simulink model "Q1b_Half_Controlled"  (R2018a)
settings: Solver=VariableStepAuto  StartTime=0.0  StopTime=1  RelTol=1e-3
libraries: powerlib x12, dspstat3 x1, powerlib_meascontrol x1
settings Model: Creator=bulbu  LastModifiedBy=bulbu

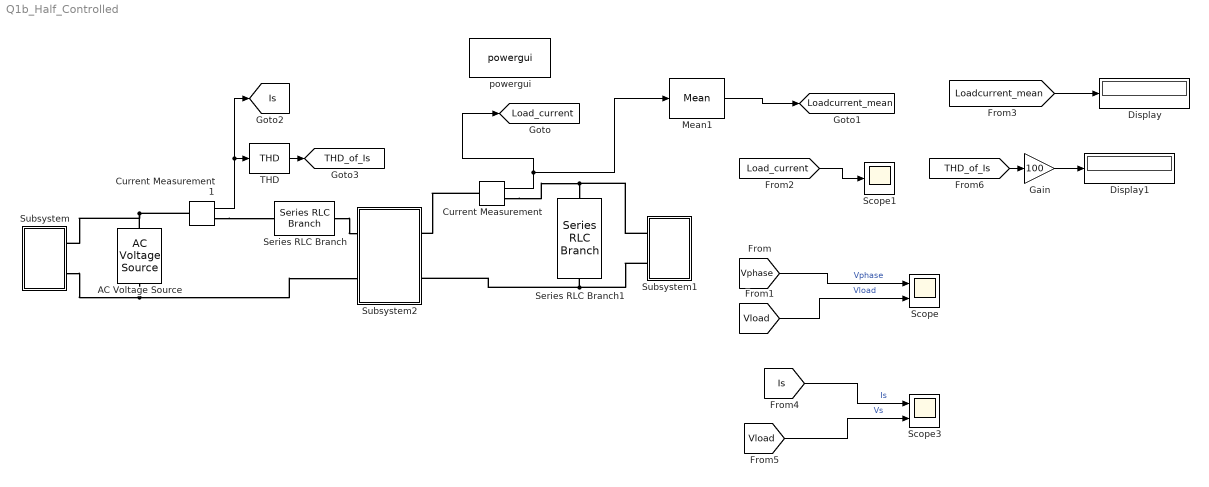
== system Q1b_Half_Controlled ==
  AC Voltage Source : powerlib/Electrical Sources/AC Voltage Source  Amplitude=326.6  Phase=0  Frequency=50  SampleTime=0  Measurements=None  BusType=swing  Pref=10e3  Qref=0  Qmin=-inf  Qmax=+inf
  Current Measurement : powerlib/Measurements/Current Measurement  PhasorSimulation=off  OutputType=Complex  PSBequivalent=0
  Current Measurement1 : powerlib/Measurements/Current Measurement  PhasorSimulation=off  OutputType=Complex  PSBequivalent=0
  Display : Display
  Display1 : Display
  Gain : Gain  Gain=100
  Mean1 : dspstat3/Mean  run=on  InputProcessing=Columns as channels (frame based)  reset_popup=None  directionMode=Each column  dimension=1  roiEnable=off  roiType=Rectangles  roiPortion=Entire ROI  roiOutput=Individual statistics for each ROI  roiFlag=off  roundingMode=Floor  overflowMode=off  outputDataTypeStr=Inherit: Same as accumulator  outputMin=[]  outputMax=[]  outputLastDataTypeStr=Inherit: Same as accumulator
  Scope : Scope  NumInputPorts=2
  Scope1 : Scope
  Scope3 : Scope  NumInputPorts=2
  Series RLC Branch : powerlib/Elements/Series RLC Branch  LConnTagsString=__new0  RConnTagsString=__new0  BranchType=L  Resistance=1  Inductance=0.5e-3  SetiL0=off  InitialCurrent=0  Capacitance=1e-6  Setx0=off  InitialVoltage=0  Measurements=None
  Series RLC Branch1 : powerlib/Elements/Series RLC Branch  LConnTagsString=__new0  RConnTagsString=__new0  BranchType=RL  Resistance=4  Inductance=200e-3  SetiL0=off  InitialCurrent=0  Capacitance=1e-6  Setx0=off  InitialVoltage=0  Measurements=None
  Subsystem : Subsystem
  Subsystem1 : Subsystem
  Subsystem2 : Subsystem
  THD : powerlib_meascontrol/Measurements/THD  Freq=50  Ts=1e-6
  powergui : powerlib/powergui  Priority=1  SimulationMode=Discrete  SampleTime=1e-6  frequency=60  Iterations=50  frequencyindice=50  Pbase=100e6  ErrMax=1e-4  UnitsV=kV  UnitsW=MW  buscounter=0  FunctionMessages=off  echomessages=off  EnableUseOfTLC=off  CurrentSourceSwitches=off  DisableSnubberDevices=off  DisableRonSwitches=off  DisableVfSwitches=off  DisplayEquations=off  SolverType=Tustin/Backward Euler (TBE)  Interpol=off  ExternalGateDelay=off  methode=off  Ts=100  x0status=blocks  SPID=on  SwTol=0  HookPort=off  RestoreLinks=warning  ResistiveCurrentMeasurement=off  Frange=[0:2:500]  Ylog=off  Xlog=on  ShowGrid=off  save=off  variable=ZData  structure=0  ZoomFFT=off  StartTime=0.0  cycles=1  DisplayStyle=1  fundamental=60  FreqAxis=off  MaxFrequency=1000  frequencyindicesteady=1  RmsSteady=1  display=off
  tag scope: Is=global, Load_current=global, Loadcurrent_mean=global, THD_of_Is=global
  wires:
  [Vload] -> Scope/2  "Vload"
  Mean1/1 -> [Loadcurrent_mean]
  [Vphase] -> Scope/1  "Vphase"
  Current Measurement/1 -> Mean1/1, [Load_current]
  [Loadcurrent_mean] -> Display/1
  [Load_current] -> Scope1/1
  Current Measurement1/1 -> [Is], THD/1
  [Is] -> Scope3/1  "Is"
  [Vload] -> Scope3/2  "Vs"
  THD/1 -> [THD_of_Is]
  [THD_of_Is] -> Gain/1
  Gain/1 -> Display1/1
  connections:
  AC Voltage Source/RConn1 -- Subsystem/LConn1 -- Current Measurement1/LConn1
  Series RLC Branch1/LConn1 -- Subsystem1/LConn1 -- Current Measurement/RConn1
  Subsystem/LConn2 -- Subsystem2/LConn2 -- AC Voltage Source/LConn1
  Subsystem1/LConn2 -- Series RLC Branch1/RConn1 -- Subsystem2/RConn2
  Current Measurement/LConn1 -- Subsystem2/RConn1
  Series RLC Branch/RConn1 -- Subsystem2/LConn1
  Current Measurement1/RConn1 -- Series RLC Branch/LConn1

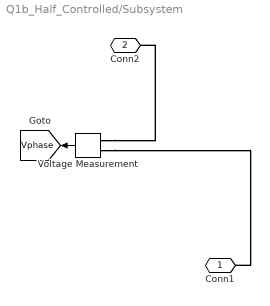
== system Q1b_Half_Controlled/Subsystem ==
  Voltage Measurement : powerlib/Measurements/Voltage Measurement  PhasorSimulation=off  OutputType=Complex  PSBequivalent=0
  Conn1 : PMIOPort  Side=Left
  Conn2 : PMIOPort  Port=2  Side=Left
  tag scope: Vphase=global
  wires:
  Voltage Measurement/1 -> [Vphase]
  connections:
  Voltage Measurement/LConn2 -- Conn2/RConn1
  Voltage Measurement/LConn1 -- Conn1/RConn1

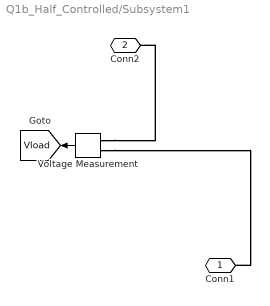
== system Q1b_Half_Controlled/Subsystem1 ==
  Voltage Measurement : powerlib/Measurements/Voltage Measurement  PhasorSimulation=off  OutputType=Complex  PSBequivalent=0
  Conn1 : PMIOPort  Side=Left
  Conn2 : PMIOPort  Port=2  Side=Left
  tag scope: Vload=global
  wires:
  Voltage Measurement/1 -> [Vload]
  connections:
  Voltage Measurement/LConn2 -- Conn2/RConn1
  Voltage Measurement/LConn1 -- Conn1/RConn1

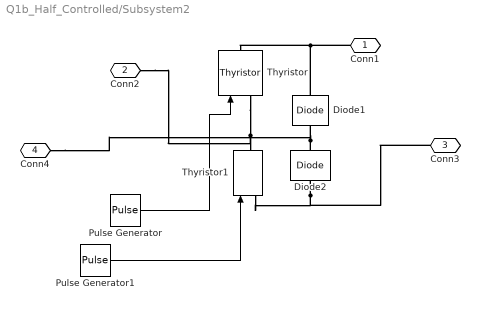
== system Q1b_Half_Controlled/Subsystem2 ==
  Diode1 : powerlib/Power Electronics/Diode  Ron=0.001  Lon=0  Vf=0.8  IC=0  UseSnubber=0  Rs=500  Cs=250e-9  Measurements=off
  Diode2 : powerlib/Power Electronics/Diode  Ron=0.001  Lon=0  Vf=0.8  IC=0  UseSnubber=0  Rs=500  Cs=250e-9  Measurements=off
  Pulse Generator : DiscretePulseGenerator  PulseType=Time based  Period=1/50  PulseWidth=50  PhaseDelay=(1/50)*(49/360)
  Pulse Generator1 : DiscretePulseGenerator  PulseType=Time based  Period=1/50  PulseWidth=50  PhaseDelay=(1/50)*(229/360)
  Thyristor : powerlib/Power Electronics/Thyristor  Ron=0.001  Lon=0  Vf=0.8  IC=0  Rs=500  Cs=250e-9  Measurements=off
  Thyristor1 : powerlib/Power Electronics/Thyristor  Ron=0.001  Lon=0  Vf=0.8  IC=0  Rs=500  Cs=250e-9  Measurements=off
  Conn1 : PMIOPort  Side=Right
  Conn2 : PMIOPort  Port=2  Side=Left
  Conn3 : PMIOPort  Port=3  Side=Right
  Conn4 : PMIOPort  Port=4  Side=Left
  wires:
  Pulse Generator1/1 -> Thyristor1/1
  Pulse Generator/1 -> Thyristor/1
  connections:
  Diode2/LConn1 -- Conn3/RConn1 -- Thyristor1/LConn1
  Diode1/RConn1 -- Conn1/RConn1 -- Thyristor/RConn1
  Diode1/LConn1 -- Conn4/RConn1 -- Diode2/RConn1
  Thyristor/LConn1 -- Conn2/RConn1 -- Thyristor1/RConn1
